simulink library "wndlib1"  (Simulink 2.09)

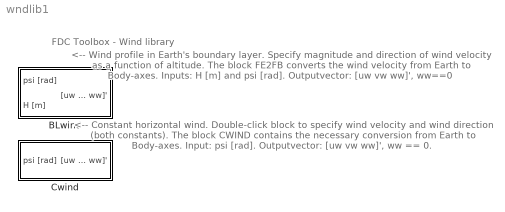
== system wndlib1 ==
  note: <-- Constant horizontal wind. Double-click block to specify wind
      | velocity and wind direction (both constants). The block CWIND
      | contains the necessary conversion from Earth to Body-axes.
      | Input: psi [rad]. Outputvector: [uw vw ww]', ww == 0.
  note: FDC Toolbox - Wind library
  note: <-- Wind profile in Earth's boundary layer. Specify magnitude and
      | direction of wind velocity as a function of altitude. The block
      | FE2FB converts the wind velocity from Earth to Body-axes.
      | Inputs: H [m] and psi [rad]. Outputvector: [uw vw ww]',  ww==0
  BLwind : Subsystem
      mask Display: disp('Windprofile in\nEarth''s boun-\ndary layer')
  Cwind : Subsystem  mask(Constant horizontal wind){Vw=15}
      mask prompts: Vw "Windspeed [m/s]:"
      mask help: Constant horizontal wind
      mask init:
      | psi_w = @2 * pi/180;
      mask Help: eval('fdchelp cwind')
      mask Display: disp('Constant hori-\nzontal wind')

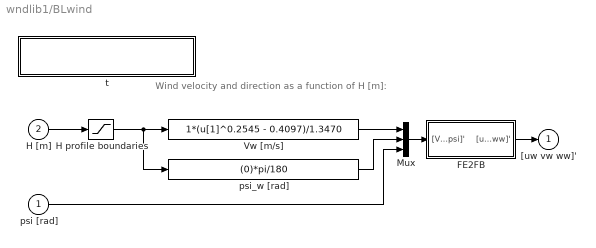
== system wndlib1/BLwind ==
  note: Wind velocity and direction
      | as a function of H [m]:
  psi [rad] : Inport  Port=1  PortWidth=-1  SampleTime=-1
  H [m] : Inport  Port=2  PortWidth=-1  SampleTime=-1
  FE2FB : Subsystem
      mask Display: disp('From Earth\nto body-axes')
  H profile boundaries : Saturate  UpperLimit=300  LowerLimit=0
  Mux : Mux  Inputs=3
  Vw [m/s] : Fcn  Expr=1*(u[1]^0.2545 - 0.4097)/1.3470
  psi_w [rad] : Fcn  Expr=(0)*pi/180
  t : Subsystem
      settings: OpenFcn=fdchelp blwind
      mask Display: disp('Wind profile in Earth''s boundary\nlayer. Marc Rauw, July 1998')
  "[uw vw ww]'" : Outport  Port=1  InitialOutput=0
  wires:
  FE2FB/1("[uw vw ww]'") -> "[uw vw ww]'"/1
  H profile boundaries/1 -> psi_w [rad]/1, Vw [m/s]/1
  H [m]/1 -> H profile boundaries/1
  Mux/1 -> FE2FB/1("[Vw psi_w psi]'")
  Vw [m/s]/1 -> Mux/1
  psi_w [rad]/1 -> Mux/2
  psi [rad]/1 -> Mux/3

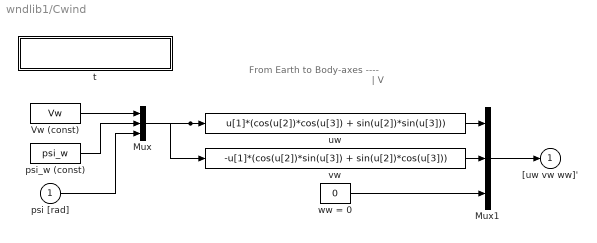
== system wndlib1/Cwind ==
  note: |
      | V
  note: From Earth to Body-axes ----
  psi [rad] : Inport  Port=1  PortWidth=-1  SampleTime=-1
  Mux : Mux  Inputs=3
  Mux1 : Mux  Inputs=3
  Vw (const) : Constant  Value=Vw
  psi_w (const) : Constant  Value=psi_w
  t : Subsystem
      settings: OpenFcn=fdchelp cwind
      mask Display: disp('Constant horizontal wind\nMarc Rauw, October 1997')
  uw : Fcn  Expr=u[1]*(cos(u[2])*cos(u[3]) + sin(u[2])*sin(u[3]))
  vw : Fcn  Expr=-u[1]*(cos(u[2])*sin(u[3]) + sin(u[2])*cos(u[3]))
  ww = 0 : Constant  Value=0
  "[uw vw ww]'" : Outport  Port=1  InitialOutput=0
  wires:
  Mux1/1 -> "[uw vw ww]'"/1
  uw/1 -> Mux1/1
  vw/1 -> Mux1/2
  ww = 0/1 -> Mux1/3
  Mux/1 -> vw/1, uw/1
  psi [rad]/1 -> Mux/3
  Vw (const)/1 -> Mux/1
  psi_w (const)/1 -> Mux/2

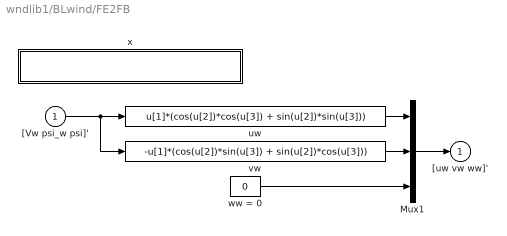
== system wndlib1/BLwind/FE2FB ==
  "[Vw psi_w psi]'" : Inport  Port=1  PortWidth=-1  SampleTime=-1
  Mux1 : Mux  Inputs=3
  uw : Fcn  Expr=u[1]*(cos(u[2])*cos(u[3]) + sin(u[2])*sin(u[3]))
  vw : Fcn  Expr=-u[1]*(cos(u[2])*sin(u[3]) + sin(u[2])*cos(u[3]))
  ww = 0 : Constant  Value=0
  x : Subsystem  Orientation=down
      mask Display: disp('Convert wind velocities from Earth\nto Body-axes. Marc Rauw, October 1997')
  "[uw vw ww]'" : Outport  Port=1  InitialOutput=0
  wires:
  "[Vw psi_w psi]'"/1 -> vw/1, uw/1
  uw/1 -> Mux1/1
  vw/1 -> Mux1/2
  ww = 0/1 -> Mux1/3
  Mux1/1 -> "[uw vw ww]'"/1

== system wndlib1/BLwind/t ==

== system wndlib1/Cwind/t ==

== system wndlib1/BLwind/FE2FB/x ==
